simulink model "C_PTES_sim_v2"  (R2025a)
settings: Solver=ode23tb  StartTime=0.0  StopTime=600
PreLoadFcn:
  | Load_Maps
InitFcn:
  | A_init_compressor
StopFcn:
  | % AB_plotHX
  | % AB_plotmap
model workspace (MAT data in the model file):
  Step_time = 1000
  step_time = 200
values from neighbouring files (symbols this model uses):
  DeltaW = 0    [A_init_compressor.m]    (also in B_init_compressor.m = input('Power change: '))
  Ki_tau = 23.1297    [A_init_compressor.m]    (also in B_init_compressor.m = 0.1)
  Kp_tau = 289.6844    [A_init_compressor.m]    (also in B_init_compressor.m = 1)
  omega_step = 376    [A_init_compressor.m]
  stepping_time = 100000    [A_init_compressor.m]    (also in B_init_compressor.m = input('Step time:'))
  tchange = 100000    [A_init_compressor.m]
undefined symbols (not defined in the file or in its folder): z_Qlty_CO2
libraries: simulink_extras x17, slpidlib x9
(part 2 of 3)

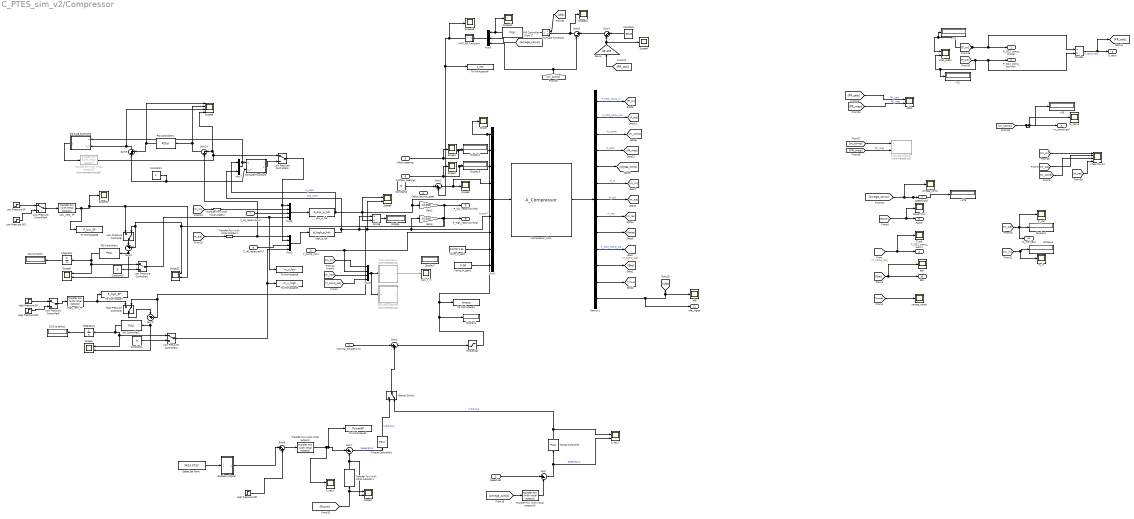
== system C_PTES_sim_v2/Compressor ==
  nominal_torque(N.m) : Inport
  Speed Set : Inport  Port=2
  T_comp_in(K) : Inport  Port=3
  Delta_recycle_open : Inport  Port=4
  Inflow_opening : Inport  Port=5
  Outflow_opening : Inport  Port=6
  T_LP_reservior(K) : Inport  Port=7
  T_HP_reservior(K) : Inport  Port=8
  CO2 to tanks : Display
  CO2 to tanks1 : Display
  Calc Inlet Temp : MATLAB Function  Commented=on  TreatAsAtomicUnit=on
  Compressor_Func : S-Function  FunctionName=A_Compressor  Parameters=Param  SFunctionDeploymentMode=off  EnableBusSupport=off
  Constant : Constant  Value=-89.45
  Constant1 : Constant
  Constant2 : Constant  Value=0
  Constant3 : Constant  Value=0
  Constant4 : Constant  Value=0
  Cool Recycle/Inlet : MATLAB Function  Commented=on  TreatAsAtomicUnit=on
  Demux1 : Demux  Outputs=13
  Display{,2..7} (7 alike) : Display
  Divide : Product  Inputs=*/
  Divide1 : Product  Inputs=/*
  Gain2 : Gain  Gain=1/1000
  Gain3 : Gain  Gain=1/1000
  Gain4 : Gain  Gain=45.455
  High Pressure Controller : ManualSwitch  CurrentSetting=0
  High Pressure SP : Step  Time=tchange  Before=7404*2.502  After=2300*2.34  SampleTime=0
  High Pressure SP1 : Step  Time=5000000  After=DeltaW  SampleTime=0
  High Pressure SP2 : Step  Time=tchange  Before=1100*2.3  After=1100*2.3  SampleTime=0
  High_vent_TF : simulink_extras/Additional Linear/Transfer Fcn (with initial outputs)  N=[1]  D=[10 1]  Y0=7404*2.502  U0=7404*2.502
  Inlet_press : Scope  NumInputPorts=2
      settings: ActiveDisplayYMinimum=-1201.3430582263272  ActiveDisplayYMaximum=21212.950352909458  DataLoggingVariableName=ScopeData18
  Integrator : Integrator
  Integrator1 : Integrator
  Low Pressure Controller : ManualSwitch  CurrentSetting=0
  Low Pressure Controller{1..5} (5 alike) : ManualSwitch
  Low Pressure SP : Step  Time=tchange  Before=7404  After=2300  SampleTime=0
  Low Pressure SP1 : Step  Time=tchange  Before=1100  After=1100  SampleTime=0
  Low_vent_TF : simulink_extras/Additional Linear/Transfer Fcn (with initial outputs)  N=[1]  D=[10 1]  Y0=7404  U0=7404
  MATLAB Function : MATLAB Function  Commented=on  TreatAsAtomicUnit=on
  MATLAB Function1 : MATLAB Function  TreatAsAtomicUnit=on
  MATLAB Function2 : MATLAB Function  TreatAsAtomicUnit=on
  MATLAB Function3 : MATLAB Function  TreatAsAtomicUnit=on
  MATLAB Function4 : MATLAB Function  TreatAsAtomicUnit=on
  Manual Switch : ManualSwitch  CurrentSetting=0
  Mux1 : Mux  Inputs=9
  Mux2 : Mux
  Mux3 : Mux
  Mux5 : Mux  Inputs=3
  Mux6 : Mux
  Mux7 : Mux  Inputs=2
  PID Controller : slpidlib/PID Controller  Controller=PI  Form=Parallel  TimeDomain=Continuous-time  UseExternalTs=off  SampleTime=-1  IntegratorMethod=Forward Euler  FilterMethod=Forward Euler  ControllerParametersSource=internal  P=0.005  I=0.0002  UseKiTs=off  D=0  UseExternalDerivativeSource=off  N=100  UseFilter=on  TunerSelectOption=Transfer Function Based (PID Tuner App)  InitialConditionSource=internal  InitialConditionForIntegrator=0  InitialConditionForFilter=0  DifferentiatorICPrevScaledInput=0  ExternalReset=none  TrackingMode=off  Kt=1  LimitOutput=on  SatLimitsSource=internal  UpperSaturationLimit=1  LowerSaturationLimit=0  LinearizeAsGain=on  AntiWindupMode=back-calculation  Kb=10  LimitIntegrator=on  UpperIntegratorSaturationLimit=inf  LowerIntegratorSaturationLimit=-inf  POutMin=[]  POutMax=[]  IOutMin=[]  IOutMax=[]  DOutMin=[]  DOutMax=[]  NOutMin=[]  NOutMax=[]  SumOutMin=[]  SumOutMax=[]  SaturationOutMin=[]  SaturationOutMax=[]  PParamMin=[]  PParamMax=[]  IParamMin=[]  IParamMax=[]  DParamMin=[]  DParamMax=[]  NParamMin=[]  NParamMax=[]  KbParamMin=[]  KbParamMax=[]  KtParamMin=[]  KtParamMax=[]  KbOutMin=[]  KbOutMax=[]  KtOutMin=[]  KtOutMax=[]  IntegratorOutMin=[]  IntegratorOutMax=[]  FilterOutMin=[]  FilterOutMax=[]  SumI1OutMin=[]  SumI1OutMax=[]  SumI2OutMin=[]  SumI2OutMax=[]  SumI3OutMin=[]  SumI3OutMax=[]  SumI4OutMin=[]  SumI4OutMax=[]  SumDOutMin=[]  SumDOutMax=[]  DifferentiatorOutMin=[]  DifferentiatorOutMax=[]  FilterDiffOutCoefMin=[]  FilterDiffOutCoefMax=[]  ReciprocalOutMin=[]  ReciprocalOutMax=[]  SumDenOutMin=[]  SumDenOutMax=[]  SumNumOutMin=[]  SumNumOutMax=[]  DivideOutMin=[]  DivideOutMax=[]  UdiffTsProdOutMin=[]  UdiffTsProdOutMax=[]  NTsProdOutMin=[]  NTsProdOutMax=[]  UintegralTsProdOutMin=[]  UintegralTsProdOutMax=[]  UngainTsProdOutMin=[]  UngainTsProdOutMax=[]  ClampingZeroOutDataTypeStr=Inherit: Inherit via back propagation  ClampingZeroOutMin=[]  ClampingZeroOutMax=[]  FilterDenConstantOutDataTypeStr=Inherit: Inherit via back propagation  FilterDenConstantOutMin=[]  FilterDenConstantOutMax=[]  PCopyOutDataTypeStr=Inherit: Inherit via back propagation  PCopyOutMin=[]  PCopyOutMax=[]  NCopyOutDataTypeStr=Inherit: Inherit via back propagation  NCopyOutMin=[]  NCopyOutMax=[]  IntegratorContinuousStateAttributes=''  IntegratorStateMustResolveToSignalObject=off  IntegratorRTWStateStorageClass=Auto  FilterContinuousStateAttributes=''  FilterStateMustResolveToSignalObject=off  FilterRTWStateStorageClass=Auto  ParallelPVariant=InternalParameters  IdealPVariant=Disabled  IVariant=InternalParameters  DVariant=Disabled  IntegratorVariant=Continuous  SatVariant=Enabled  AWVariant=BackCalculation  PCopyVariant=Disabled  TRVariant=Disabled  FdbkBlocksVariant=Forward  IdealPFdbkVariant=Disabled  SatFdbkVariant=Disabled  DerivativeFilterVariant=Disabled  NVariant=Disabled  NCopyVariant=Disabled_SignalSpec  FilterICVariant=Disabled  IntegratorICVariant=InternalICs  ExternalResetVariant=Disabled  TRSumVariant=Passthrough  SumFdbkVariant=Disabled  SumVariant=Sum_PI  TsampFilterVariant=InternalTs  TsampNgainVariant=Passthrough  TsampIntegralVariant=Disabled_SignalSpec  ExternalSaturationOutDataTypeStr=Inherit: Same as second input  DerivativeSourceVariant=Disabled  PreIntVariant=InternalPreInt
  PID Controller1 : slpidlib/PID Controller  Controller=PI  Form=Parallel  TimeDomain=Continuous-time  UseExternalTs=off  SampleTime=-1  IntegratorMethod=Forward Euler  FilterMethod=Forward Euler  ControllerParametersSource=internal  P=0.005  I=0.003  UseKiTs=off  D=0  UseExternalDerivativeSource=off  N=100  UseFilter=on  TunerSelectOption=Transfer Function Based (PID Tuner App)  InitialConditionSource=internal  InitialConditionForIntegrator=0  InitialConditionForFilter=0  DifferentiatorICPrevScaledInput=0  ExternalReset=none  TrackingMode=off  Kt=1  LimitOutput=off  SatLimitsSource=internal  UpperSaturationLimit=50  LowerSaturationLimit=-50  LinearizeAsGain=on  AntiWindupMode=none  Kb=1  LimitIntegrator=off  UpperIntegratorSaturationLimit=inf  LowerIntegratorSaturationLimit=-inf  POutMin=[]  POutMax=[]  IOutMin=[]  IOutMax=[]  DOutMin=[]  DOutMax=[]  NOutMin=[]  NOutMax=[]  SumOutMin=[]  SumOutMax=[]  SaturationOutMin=[]  SaturationOutMax=[]  PParamMin=[]  PParamMax=[]  IParamMin=[]  IParamMax=[]  DParamMin=[]  DParamMax=[]  NParamMin=[]  NParamMax=[]  KbParamMin=[]  KbParamMax=[]  KtParamMin=[]  KtParamMax=[]  KbOutMin=[]  KbOutMax=[]  KtOutMin=[]  KtOutMax=[]  IntegratorOutMin=[]  IntegratorOutMax=[]  FilterOutMin=[]  FilterOutMax=[]  SumI1OutMin=[]  SumI1OutMax=[]  SumI2OutMin=[]  SumI2OutMax=[]  SumI3OutMin=[]  SumI3OutMax=[]  SumI4OutMin=[]  SumI4OutMax=[]  SumDOutMin=[]  SumDOutMax=[]  DifferentiatorOutMin=[]  DifferentiatorOutMax=[]  FilterDiffOutCoefMin=[]  FilterDiffOutCoefMax=[]  ReciprocalOutMin=[]  ReciprocalOutMax=[]  SumDenOutMin=[]  SumDenOutMax=[]  SumNumOutMin=[]  SumNumOutMax=[]  DivideOutMin=[]  DivideOutMax=[]  UdiffTsProdOutMin=[]  UdiffTsProdOutMax=[]  NTsProdOutMin=[]  NTsProdOutMax=[]  UintegralTsProdOutMin=[]  UintegralTsProdOutMax=[]  UngainTsProdOutMin=[]  UngainTsProdOutMax=[]  ClampingZeroOutDataTypeStr=Inherit: Inherit via back propagation  ClampingZeroOutMin=[]  ClampingZeroOutMax=[]  FilterDenConstantOutDataTypeStr=Inherit: Inherit via back propagation  FilterDenConstantOutMin=[]  FilterDenConstantOutMax=[]  PCopyOutDataTypeStr=Inherit: Inherit via back propagation  PCopyOutMin=[]  PCopyOutMax=[]  NCopyOutDataTypeStr=Inherit: Inherit via back propagation  NCopyOutMin=[]  NCopyOutMax=[]  IntegratorContinuousStateAttributes=''  IntegratorStateMustResolveToSignalObject=off  IntegratorRTWStateStorageClass=Auto  FilterContinuousStateAttributes=''  FilterStateMustResolveToSignalObject=off  FilterRTWStateStorageClass=Auto  ParallelPVariant=InternalParameters  IdealPVariant=Disabled  IVariant=InternalParameters  DVariant=Disabled  IntegratorVariant=Continuous  SatVariant=Disabled  AWVariant=Passthrough  PCopyVariant=Disabled  TRVariant=Disabled  FdbkBlocksVariant=Forward  IdealPFdbkVariant=Disabled  SatFdbkVariant=Disabled  DerivativeFilterVariant=Disabled  NVariant=Disabled  NCopyVariant=Disabled_SignalSpec  FilterICVariant=Disabled  IntegratorICVariant=InternalICs  ExternalResetVariant=Disabled  TRSumVariant=Passthrough  SumFdbkVariant=Disabled  SumVariant=Sum_PI  TsampFilterVariant=InternalTs  TsampNgainVariant=Passthrough  TsampIntegralVariant=Disabled_SignalSpec  ExternalSaturationOutDataTypeStr=Inherit: Same as second input  DerivativeSourceVariant=Disabled  PreIntVariant=InternalPreInt
  PID Controller2 : slpidlib/PID Controller  Controller=PI  Form=Parallel  TimeDomain=Continuous-time  UseExternalTs=off  SampleTime=-1  IntegratorMethod=Forward Euler  FilterMethod=Forward Euler  ControllerParametersSource=internal  P=0.005  I=0.003  UseKiTs=off  D=0  UseExternalDerivativeSource=off  N=100  UseFilter=on  TunerSelectOption=Transfer Function Based (PID Tuner App)  InitialConditionSource=internal  InitialConditionForIntegrator=0  InitialConditionForFilter=0  DifferentiatorICPrevScaledInput=0  ExternalReset=none  TrackingMode=off  Kt=1  LimitOutput=off  SatLimitsSource=internal  UpperSaturationLimit=50  LowerSaturationLimit=-50  LinearizeAsGain=on  AntiWindupMode=back-calculation  Kb=1  LimitIntegrator=off  UpperIntegratorSaturationLimit=inf  LowerIntegratorSaturationLimit=-inf  POutMin=[]  POutMax=[]  IOutMin=[]  IOutMax=[]  DOutMin=[]  DOutMax=[]  NOutMin=[]  NOutMax=[]  SumOutMin=[]  SumOutMax=[]  SaturationOutMin=[]  SaturationOutMax=[]  PParamMin=[]  PParamMax=[]  IParamMin=[]  IParamMax=[]  DParamMin=[]  DParamMax=[]  NParamMin=[]  NParamMax=[]  KbParamMin=[]  KbParamMax=[]  KtParamMin=[]  KtParamMax=[]  KbOutMin=[]  KbOutMax=[]  KtOutMin=[]  KtOutMax=[]  IntegratorOutMin=[]  IntegratorOutMax=[]  FilterOutMin=[]  FilterOutMax=[]  SumI1OutMin=[]  SumI1OutMax=[]  SumI2OutMin=[]  SumI2OutMax=[]  SumI3OutMin=[]  SumI3OutMax=[]  SumI4OutMin=[]  SumI4OutMax=[]  SumDOutMin=[]  SumDOutMax=[]  DifferentiatorOutMin=[]  DifferentiatorOutMax=[]  FilterDiffOutCoefMin=[]  FilterDiffOutCoefMax=[]  ReciprocalOutMin=[]  ReciprocalOutMax=[]  SumDenOutMin=[]  SumDenOutMax=[]  SumNumOutMin=[]  SumNumOutMax=[]  DivideOutMin=[]  DivideOutMax=[]  UdiffTsProdOutMin=[]  UdiffTsProdOutMax=[]  NTsProdOutMin=[]  NTsProdOutMax=[]  UintegralTsProdOutMin=[]  UintegralTsProdOutMax=[]  UngainTsProdOutMin=[]  UngainTsProdOutMax=[]  ClampingZeroOutDataTypeStr=Inherit: Inherit via back propagation  ClampingZeroOutMin=[]  ClampingZeroOutMax=[]  FilterDenConstantOutDataTypeStr=Inherit: Inherit via back propagation  FilterDenConstantOutMin=[]  FilterDenConstantOutMax=[]  PCopyOutDataTypeStr=Inherit: Inherit via back propagation  PCopyOutMin=[]  PCopyOutMax=[]  NCopyOutDataTypeStr=Inherit: Inherit via back propagation  NCopyOutMin=[]  NCopyOutMax=[]  IntegratorContinuousStateAttributes=''  IntegratorStateMustResolveToSignalObject=off  IntegratorRTWStateStorageClass=Auto  FilterContinuousStateAttributes=''  FilterStateMustResolveToSignalObject=off  FilterRTWStateStorageClass=Auto  ParallelPVariant=InternalParameters  IdealPVariant=Disabled  IVariant=InternalParameters  DVariant=Disabled  IntegratorVariant=Continuous  SatVariant=Disabled  AWVariant=Passthrough  PCopyVariant=Disabled  TRVariant=Disabled  FdbkBlocksVariant=Forward  IdealPFdbkVariant=Disabled  SatFdbkVariant=Disabled  DerivativeFilterVariant=Disabled  NVariant=Disabled  NCopyVariant=Disabled_SignalSpec  FilterICVariant=Disabled  IntegratorICVariant=InternalICs  ExternalResetVariant=Disabled  TRSumVariant=Passthrough  SumFdbkVariant=Disabled  SumVariant=Sum_PI  TsampFilterVariant=InternalTs  TsampNgainVariant=Passthrough  TsampIntegralVariant=Disabled_SignalSpec  ExternalSaturationOutDataTypeStr=Inherit: Same as second input  DerivativeSourceVariant=Disabled  PreIntVariant=InternalPreInt
  PID Controller3 : slpidlib/PID Controller  Controller=PID  Form=Parallel  TimeDomain=Continuous-time  UseExternalTs=off  SampleTime=-1  IntegratorMethod=Forward Euler  FilterMethod=Forward Euler  ControllerParametersSource=internal  P=2  I=0.5  UseKiTs=off  D=0  UseExternalDerivativeSource=off  N=100  UseFilter=on  TunerSelectOption=Transfer Function Based (PID Tuner App)  InitialConditionSource=internal  InitialConditionForIntegrator=0  InitialConditionForFilter=0  DifferentiatorICPrevScaledInput=0  ExternalReset=none  TrackingMode=off  Kt=1  LimitOutput=on  SatLimitsSource=internal  UpperSaturationLimit=5  LowerSaturationLimit=-1  LinearizeAsGain=on  AntiWindupMode=back-calculation  Kb=1  LimitIntegrator=off  UpperIntegratorSaturationLimit=inf  LowerIntegratorSaturationLimit=-inf  POutMin=[]  POutMax=[]  IOutMin=[]  IOutMax=[]  DOutMin=[]  DOutMax=[]  NOutMin=[]  NOutMax=[]  SumOutMin=[]  SumOutMax=[]  SaturationOutMin=[]  SaturationOutMax=[]  PParamMin=[]  PParamMax=[]  IParamMin=[]  IParamMax=[]  DParamMin=[]  DParamMax=[]  NParamMin=[]  NParamMax=[]  KbParamMin=[]  KbParamMax=[]  KtParamMin=[]  KtParamMax=[]  KbOutMin=[]  KbOutMax=[]  KtOutMin=[]  KtOutMax=[]  IntegratorOutMin=[]  IntegratorOutMax=[]  FilterOutMin=[]  FilterOutMax=[]  SumI1OutMin=[]  SumI1OutMax=[]  SumI2OutMin=[]  SumI2OutMax=[]  SumI3OutMin=[]  SumI3OutMax=[]  SumI4OutMin=[]  SumI4OutMax=[]  SumDOutMin=[]  SumDOutMax=[]  DifferentiatorOutMin=[]  DifferentiatorOutMax=[]  FilterDiffOutCoefMin=[]  FilterDiffOutCoefMax=[]  ReciprocalOutMin=[]  ReciprocalOutMax=[]  SumDenOutMin=[]  SumDenOutMax=[]  SumNumOutMin=[]  SumNumOutMax=[]  DivideOutMin=[]  DivideOutMax=[]  UdiffTsProdOutMin=[]  UdiffTsProdOutMax=[]  NTsProdOutMin=[]  NTsProdOutMax=[]  UintegralTsProdOutMin=[]  UintegralTsProdOutMax=[]  UngainTsProdOutMin=[]  UngainTsProdOutMax=[]  ClampingZeroOutDataTypeStr=Inherit: Inherit via back propagation  ClampingZeroOutMin=[]  ClampingZeroOutMax=[]  FilterDenConstantOutDataTypeStr=Inherit: Inherit via back propagation  FilterDenConstantOutMin=[]  FilterDenConstantOutMax=[]  PCopyOutDataTypeStr=Inherit: Inherit via back propagation  PCopyOutMin=[]  PCopyOutMax=[]  NCopyOutDataTypeStr=Inherit: Inherit via back propagation  NCopyOutMin=[]  NCopyOutMax=[]  IntegratorContinuousStateAttributes=''  IntegratorStateMustResolveToSignalObject=off  IntegratorRTWStateStorageClass=Auto  FilterContinuousStateAttributes=''  FilterStateMustResolveToSignalObject=off  FilterRTWStateStorageClass=Auto  ParallelPVariant=InternalParameters  IdealPVariant=Disabled  IVariant=InternalParameters  DVariant=InternalParameters  IntegratorVariant=Continuous  SatVariant=Enabled  AWVariant=BackCalculation  PCopyVariant=Disabled  TRVariant=Disabled  FdbkBlocksVariant=Forward  IdealPFdbkVariant=Disabled  SatFdbkVariant=Disabled  DerivativeFilterVariant=ContFilter  NVariant=InternalParameters  NCopyVariant=Disabled  FilterICVariant=InternalICsFilter  IntegratorICVariant=InternalICs  ExternalResetVariant=Disabled  TRSumVariant=Passthrough  SumFdbkVariant=Disabled  SumVariant=Sum_PID  TsampFilterVariant=InternalTs  TsampNgainVariant=Passthrough  TsampIntegralVariant=Disabled_SignalSpec  ExternalSaturationOutDataTypeStr=Inherit: Same as second input  DerivativeSourceVariant=ErrorSignal  PreIntVariant=InternalPreInt
  Power(kW) : Scope
      settings: ActiveDisplayYMinimum=9621.7825106762266  ActiveDisplayYMaximum=9623.07314717155  DataLoggingSaveFormat=Array
  Scope{,1..3,9..11,13..14} (9 alike) : Scope
      Scope settings: ActiveDisplayYMinimum=7159.4982132893756  ActiveDisplayYMaximum=32715.546490584897  DataLoggingVariableName=ScopeData2
      Scope1 settings: ActiveDisplayYMinimum=0.66249029672546578  ActiveDisplayYMaximum=1.037501078141615  DataLoggingVariableName=ScopeData3
      Scope10 settings: ActiveDisplayYMinimum=-0.1487440658614268  ActiveDisplayYMaximum=0.0708941770326301  DataLoggingVariableName=ScopeData2
      Scope11 settings: ActiveDisplayYMinimum=-1  ActiveDisplayYMaximum=1  DataLoggingVariableName=ScopeData3
      Scope13 settings: ActiveDisplayYMinimum=7403.9999999999982  ActiveDisplayYMaximum=7404.0000000000036  DataLoggingVariableName=ScopeData63
      Scope14 settings: ActiveDisplayYMinimum=-62.947751511362974  ActiveDisplayYMaximum=-19.709497965627289  DataLoggingVariableName=ScopeData86
      Scope2 settings: ActiveDisplayYMinimum=0.43749999999999889  ActiveDisplayYMaximum=1.0625000000000007  DataLoggingVariableName=ScopeData4
      Scope3 settings: ActiveDisplayYMinimum=-4.9775352924503617E-5  ActiveDisplayYMaximum=2.2984047573706729E-5  DataLoggingVariableName=ScopeData4
      Scope9 settings: ActiveDisplayYMinimum=34.362516239027393  ActiveDisplayYMaximum=130.4282542390518
  Scope{4..7,12} (5 alike) : Scope  NumInputPorts=2
      Scope12 settings: ActiveDisplayYMinimum=5734.2862269607867  ActiveDisplayYMaximum=17518.250083003895  DataLoggingVariableName=ScopeData41
      Scope4 settings: ActiveDisplayYMinimum=-0.00074119709145113429  ActiveDisplayYMaximum=0.0001840673230964241  DataLoggingVariableName=ScopeData20
      Scope5 settings: ActiveDisplayYMinimum=-1  ActiveDisplayYMaximum=1  DataLoggingVariableName=ScopeData43
      Scope6 settings: ActiveDisplayYMinimum=-1.078293953241016E+6  ActiveDisplayYMaximum=2.0704645579169132E+7
      Scope7 settings: ActiveDisplayYMinimum=9621.7825106762266  ActiveDisplayYMaximum=9623.07314717155  DataLoggingVariableName=ScopeData7
  Scope8 : Scope  NumInputPorts=4
      settings: ActiveDisplayYMinimum=-2.4702730991182236  ActiveDisplayYMaximum=3.070460845323943  DataLoggingVariableName=ScopeData88
  Shutdown Signal : Subsystem
  Speed Set Point : Constant  Value=9623.0732
  Sum : Sum  Inputs=|+-
  Sum{1..2,5,8..9} (5 alike) : Sum  Inputs=|++
  Sum10 : Sum  Inputs=|-+
  Sum3 : Sum  Inputs=|-+
  Sum4 : Sum  Inputs=|-+
  Sum6 : Sum  Inputs=|+-
  Sum7 : Sum  Inputs=|+-
  T_out : Scope
      settings: ActiveDisplayYMinimum=840.98204874336943  ActiveDisplayYMaximum=841.08678779671368  DataLoggingVariableName=ScopeData11  DataLoggingSaveFormat=Array
  To Workspace1 : ToWorkspace  VariableName=torque  SampleTime=-1
      settings: Save2DSignal=2-D array (concatenate along first dimension)
  To Workspace2 : ToWorkspace  VariableName=PowerSP  SampleTime=-1
      settings: Save2DSignal=2-D array (concatenate along first dimension)
  To Workspace3 : ToWorkspace  VariableName=m_v_low  SampleTime=-1
      settings: Save2DSignal=2-D array (concatenate along first dimension)
  To Workspace4 : ToWorkspace  VariableName=z_rec  SampleTime=-1
      settings: Save2DSignal=2-D array (concatenate along first dimension)
  To Workspace5 : ToWorkspace  VariableName=m_v_high  SampleTime=-1
      settings: Save2DSignal=2-D array (concatenate along first dimension)
  To Workspace6 : ToWorkspace  VariableName=P_low_SP  SampleTime=-1
      settings: Save2DSignal=2-D array (concatenate along first dimension)
  To Workspace7 : ToWorkspace  VariableName=P_high_SP  SampleTime=-1
      settings: Save2DSignal=2-D array (concatenate along first dimension)
  Torque Controller : slpidlib/PID Controller  Controller=PI  Form=Parallel  TimeDomain=Continuous-time  UseExternalTs=off  SampleTime=-1  IntegratorMethod=Forward Euler  FilterMethod=Forward Euler  ControllerParametersSource=internal  P=Kp_tau  I=Ki_tau  UseKiTs=off  D=0  UseExternalDerivativeSource=off  N=100  UseFilter=on  TunerSelectOption=Transfer Function Based (PID Tuner App)  InitialConditionSource=internal  InitialConditionForIntegrator=0  InitialConditionForFilter=0  DifferentiatorICPrevScaledInput=0  ExternalReset=none  TrackingMode=off  Kt=1  LimitOutput=off  SatLimitsSource=internal  UpperSaturationLimit=inf  LowerSaturationLimit=-inf  LinearizeAsGain=on  AntiWindupMode=none  Kb=1  LimitIntegrator=off  UpperIntegratorSaturationLimit=inf  LowerIntegratorSaturationLimit=-inf  POutMin=[]  POutMax=[]  IOutMin=[]  IOutMax=[]  DOutMin=[]  DOutMax=[]  NOutMin=[]  NOutMax=[]  SumOutMin=[]  SumOutMax=[]  SaturationOutMin=[]  SaturationOutMax=[]  PParamMin=[]  PParamMax=[]  IParamMin=[]  IParamMax=[]  DParamMin=[]  DParamMax=[]  NParamMin=[]  NParamMax=[]  KbParamMin=[]  KbParamMax=[]  KtParamMin=[]  KtParamMax=[]  KbOutMin=[]  KbOutMax=[]  KtOutMin=[]  KtOutMax=[]  IntegratorOutMin=[]  IntegratorOutMax=[]  FilterOutMin=[]  FilterOutMax=[]  SumI1OutMin=[]  SumI1OutMax=[]  SumI2OutMin=[]  SumI2OutMax=[]  SumI3OutMin=[]  SumI3OutMax=[]  SumI4OutMin=[]  SumI4OutMax=[]  SumDOutMin=[]  SumDOutMax=[]  DifferentiatorOutMin=[]  DifferentiatorOutMax=[]  FilterDiffOutCoefMin=[]  FilterDiffOutCoefMax=[]  ReciprocalOutMin=[]  ReciprocalOutMax=[]  SumDenOutMin=[]  SumDenOutMax=[]  SumNumOutMin=[]  SumNumOutMax=[]  DivideOutMin=[]  DivideOutMax=[]  UdiffTsProdOutMin=[]  UdiffTsProdOutMax=[]  NTsProdOutMin=[]  NTsProdOutMax=[]  UintegralTsProdOutMin=[]  UintegralTsProdOutMax=[]  UngainTsProdOutMin=[]  UngainTsProdOutMax=[]  ClampingZeroOutDataTypeStr=Inherit: Inherit via back propagation  ClampingZeroOutMin=[]  ClampingZeroOutMax=[]  FilterDenConstantOutDataTypeStr=Inherit: Inherit via back propagation  FilterDenConstantOutMin=[]  FilterDenConstantOutMax=[]  PCopyOutDataTypeStr=Inherit: Inherit via back propagation  PCopyOutMin=[]  PCopyOutMax=[]  NCopyOutDataTypeStr=Inherit: Inherit via back propagation  NCopyOutMin=[]  NCopyOutMax=[]  IntegratorContinuousStateAttributes=''  IntegratorStateMustResolveToSignalObject=off  IntegratorRTWStateStorageClass=Auto  FilterContinuousStateAttributes=''  FilterStateMustResolveToSignalObject=off  FilterRTWStateStorageClass=Auto  ParallelPVariant=InternalParameters  IdealPVariant=Disabled  IVariant=InternalParameters  DVariant=Disabled  IntegratorVariant=Continuous  SatVariant=Disabled  AWVariant=Passthrough  PCopyVariant=Disabled  TRVariant=Disabled  FdbkBlocksVariant=Forward  IdealPFdbkVariant=Disabled  SatFdbkVariant=Disabled  DerivativeFilterVariant=Disabled  NVariant=Disabled  NCopyVariant=Disabled_SignalSpec  FilterICVariant=Disabled  IntegratorICVariant=InternalICs  ExternalResetVariant=Disabled  TRSumVariant=Passthrough  SumFdbkVariant=Disabled  SumVariant=Sum_PI  TsampFilterVariant=InternalTs  TsampNgainVariant=Passthrough  TsampIntegralVariant=Disabled_SignalSpec  ExternalSaturationOutDataTypeStr=Inherit: Same as second input  DerivativeSourceVariant=Disabled  PreIntVariant=InternalPreInt
  Torque Controller1 : slpidlib/PID Controller  Controller=PI  Form=Parallel  TimeDomain=Continuous-time  UseExternalTs=off  SampleTime=-1  IntegratorMethod=Forward Euler  FilterMethod=Forward Euler  ControllerParametersSource=internal  P=0.16  I=0.09  UseKiTs=off  D=0  UseExternalDerivativeSource=off  N=100  UseFilter=on  TunerSelectOption=Transfer Function Based (PID Tuner App)  InitialConditionSource=internal  InitialConditionForIntegrator=3.258241730106488e+04  InitialConditionForFilter=0  DifferentiatorICPrevScaledInput=0  ExternalReset=none  TrackingMode=off  Kt=1  LimitOutput=off  SatLimitsSource=internal  UpperSaturationLimit=inf  LowerSaturationLimit=-inf  LinearizeAsGain=on  AntiWindupMode=none  Kb=1  LimitIntegrator=off  UpperIntegratorSaturationLimit=inf  LowerIntegratorSaturationLimit=-inf  POutMin=[]  POutMax=[]  IOutMin=[]  IOutMax=[]  DOutMin=[]  DOutMax=[]  NOutMin=[]  NOutMax=[]  SumOutMin=[]  SumOutMax=[]  SaturationOutMin=[]  SaturationOutMax=[]  PParamMin=[]  PParamMax=[]  IParamMin=[]  IParamMax=[]  DParamMin=[]  DParamMax=[]  NParamMin=[]  NParamMax=[]  KbParamMin=[]  KbParamMax=[]  KtParamMin=[]  KtParamMax=[]  KbOutMin=[]  KbOutMax=[]  KtOutMin=[]  KtOutMax=[]  IntegratorOutMin=[]  IntegratorOutMax=[]  FilterOutMin=[]  FilterOutMax=[]  SumI1OutMin=[]  SumI1OutMax=[]  SumI2OutMin=[]  SumI2OutMax=[]  SumI3OutMin=[]  SumI3OutMax=[]  SumI4OutMin=[]  SumI4OutMax=[]  SumDOutMin=[]  SumDOutMax=[]  DifferentiatorOutMin=[]  DifferentiatorOutMax=[]  FilterDiffOutCoefMin=[]  FilterDiffOutCoefMax=[]  ReciprocalOutMin=[]  ReciprocalOutMax=[]  SumDenOutMin=[]  SumDenOutMax=[]  SumNumOutMin=[]  SumNumOutMax=[]  DivideOutMin=[]  DivideOutMax=[]  UdiffTsProdOutMin=[]  UdiffTsProdOutMax=[]  NTsProdOutMin=[]  NTsProdOutMax=[]  UintegralTsProdOutMin=[]  UintegralTsProdOutMax=[]  UngainTsProdOutMin=[]  UngainTsProdOutMax=[]  ClampingZeroOutDataTypeStr=Inherit: Inherit via back propagation  ClampingZeroOutMin=[]  ClampingZeroOutMax=[]  FilterDenConstantOutDataTypeStr=Inherit: Inherit via back propagation  FilterDenConstantOutMin=[]  FilterDenConstantOutMax=[]  PCopyOutDataTypeStr=Inherit: Inherit via back propagation  PCopyOutMin=[]  PCopyOutMax=[]  NCopyOutDataTypeStr=Inherit: Inherit via back propagation  NCopyOutMin=[]  NCopyOutMax=[]  IntegratorContinuousStateAttributes=''  IntegratorStateMustResolveToSignalObject=off  IntegratorRTWStateStorageClass=Auto  FilterContinuousStateAttributes=''  FilterStateMustResolveToSignalObject=off  FilterRTWStateStorageClass=Auto  ParallelPVariant=InternalParameters  IdealPVariant=Disabled  IVariant=InternalParameters  DVariant=Disabled  IntegratorVariant=Continuous  SatVariant=Disabled  AWVariant=Passthrough  PCopyVariant=Disabled  TRVariant=Disabled  FdbkBlocksVariant=Forward  IdealPFdbkVariant=Disabled  SatFdbkVariant=Disabled  DerivativeFilterVariant=Disabled  NVariant=Disabled  NCopyVariant=Disabled_SignalSpec  FilterICVariant=Disabled  IntegratorICVariant=InternalICs  ExternalResetVariant=Disabled  TRSumVariant=Passthrough  SumFdbkVariant=Disabled  SumVariant=Sum_PI  TsampFilterVariant=InternalTs  TsampNgainVariant=Passthrough  TsampIntegralVariant=Disabled_SignalSpec  ExternalSaturationOutDataTypeStr=Inherit: Same as second input  DerivativeSourceVariant=Disabled  PreIntVariant=InternalPreInt
  Torque Sat : Saturate  UpperLimit=4.2570e4  LowerLimit=0
  Transfer Fcn (with initial outputs) : simulink_extras/Additional Linear/Transfer Fcn (with initial outputs)  N=[1]  D="[1  1]"  Y0=9623.0732  U0=0
  Transfer Fcn (with initial outputs)1 : simulink_extras/Additional Linear/Transfer Fcn (with initial outputs)  N=[1]  D="[1  1]"  Y0=9623.0732  U0=0
  Transfer Fcn (with initial outputs)2 : simulink_extras/Additional Linear/Transfer Fcn (with initial outputs)  Commented=through  N=[1]  D="[1  1]"  Y0=53.3769  U0=0
  Transfer Fcn (with initial outputs)3 : simulink_extras/Additional Linear/Transfer Fcn (with initial outputs)  N=[1]  D="[1  1]"  Y0=376  U0=0
  Transfer Fcn (with initial states) : simulink_extras/Additional Linear/Transfer Fcn (with initial states)  N=[1]  D="[1  1]"  X0=53.0908043651412
  Transfer Fcn (with initial states)1 : simulink_extras/Additional Linear/Transfer Fcn (with initial states)  N=[1]  D="[1  1]"  X0=53.0908043651412
  Valve_in_gain : Constant  Value=0.1071*1.34
  Valve_in_gain1 : Constant  Value=0.08
  calc_t_in : Scope
      settings: ActiveDisplayYMinimum=-1  ActiveDisplayYMaximum=1  DataLoggingVariableName=ScopeData22  DataLoggingSaveFormat=Array
  eta : Scope
      settings: ActiveDisplayYMinimum=0.058346045029937676  ActiveDisplayYMaximum=0.974885594730561  DataLoggingVariableName=ScopeData12  DataLoggingSaveFormat=Array
  high_p_hdr : S-Function  FunctionName=A_high_p_hdr  Parameters=Param  SFunctionDeploymentMode=off  EnableBusSupport=off
  idle : Scope
      settings: ActiveDisplayYMinimum=-0.12499999999999997  ActiveDisplayYMaximum=1.125  DataLoggingVariableName=ScopeData21  DataLoggingSaveFormat=Array
  idle1 : Scope  NumInputPorts=2
      settings: ActiveDisplayYMinimum=0.94027654878005018  ActiveDisplayYMaximum=1.1257908746996972  DataLoggingVariableName=ScopeData40
  low_p_hdr : S-Function  FunctionName=A_low_p_hdr  Parameters=Param  SFunctionDeploymentMode=off  EnableBusSupport=off
  m_comp : Scope
      settings: ActiveDisplayYMinimum=-6.4294152227829491  ActiveDisplayYMaximum=57.864737008156951  DataLoggingVariableName=ScopeData13  DataLoggingSaveFormat=Array
  m_in : Scope
      settings: ActiveDisplayYMinimum=-5.7642251489523835  ActiveDisplayYMaximum=51.878026340571459  DataLoggingVariableName=ScopeData14
  m_out : Scope
      settings: ActiveDisplayYMinimum=-1.9413639664669944  ActiveDisplayYMaximum=2.9528309069791945  DataLoggingVariableName=ScopeData2
  mass flows1 : Scope  NumInputPorts=4
      settings: ActiveDisplayYMinimum=-6.6752308438687669  ActiveDisplayYMaximum=60.077077594818917  DataLoggingVariableName=ScopeData16  DataLoggingSaveFormat=Array
  omega_comp : Scope
      settings: ActiveDisplayYMinimum=8.3712039774254627  ActiveDisplayYMaximum=10.897406611126089  DataLoggingVariableName=ScopeData17
  t_rec1 : Scope  NumInputPorts=2
      settings: ActiveDisplayYMinimum=-0.00059724971531247353  ActiveDisplayYMaximum=0.00016704312745400825  DataLoggingVariableName=ScopeData87  DataLoggingSaveFormat=Array
  t_rec2 : Scope  NumInputPorts=2
      settings: ActiveDisplayYMinimum=-1202.88415  ActiveDisplayYMaximum=10825.957350000002  DataLoggingVariableName=ScopeData24  DataLoggingSaveFormat=Array
  torque_comp : Scope
      settings: ActiveDisplayYMinimum=-3437.51384  ActiveDisplayYMaximum=30937.62455  DataLoggingSaveFormat=Array
  ~22 : Display
  ~379 : Display
  ~55 : Display
  ~7.4 : Display
  P_CO2_comp_in(kPa) : Outport
  P_CO2_comp_out(kPa) : Outport  Port=2
  m_comp(kg/s) : Outport  Port=3
  T_CO2_comp_out(K) : Outport  Port=4
  P_low_reservior(kPa) : Outport  Port=5
  P_high_reservior(kPa) : Outport  Port=6
  Speed(rpm) : Outport  Port=7
  P_ratio : Outport  Port=8
  Power : Outport  Port=9
  Eta : Outport  Port=10
  idle_signal : Outport  Port=11
  m_out(kg/s) : Outport  Port=12
  wires:
  Demux1/10 -> [T_comp_out]  "T_CO2_comp_out"
  Demux1/12 -> [Torque]
  Demux1/6 -> [m_in]  "M_in"
  Demux1/3 -> [m_comp]  "M_comp"
  Demux1/2 -> [P_out]  "P_CO2_comp_out"
  Compressor_Func/1 -> Demux1/1
  Demux1/8 -> [m_rec]  "m_rec"
  Demux1/1 -> [P_in]  "P_CO2_comp_in"
  Demux1/11 -> [Eta]
  Demux1/9 -> [Power]
  Sum/1 -> t_rec1/2, Torque Controller/1  "Speed Error"
  Mux1/1 -> Compressor_Func/1
  Divide/1 -> Display/1
  Mux3/1 -> low_p_hdr/1
  Mux2/1 -> high_p_hdr/1
  Demux1/5 -> [omega_comp]
  Transfer Fcn (with initial states)/1 -> Mux3/2
  Transfer Fcn (with initial states)1/1 -> Sum10/2, Mux2/1
  Gain2/1 -> Low Pressure Controller/2, Sum4/2, Scope12/1, P_low_reservior(kPa)/1
  Demux1/4 -> [PR_map]  "P_ratio"
  Sum2/1 -> Scope3/1, Mux1/4
  Inflow_opening/1 -> Scope1/1, Display2/1, Mux1/2
  Outflow_opening/1 -> Scope2/1, Display3/1, Mux1/3
  T_HP_reservior(K)/1 -> Mux2/3
  T_LP_reservior(K)/1 -> Mux3/3
  Constant/1 -> Sum5/1
  Sum5/1 -> Sum6/1
  Sum6/1 -> MATLAB Function2/2(x), Scope14/1
  Demux1/7 -> [m_out]  "M_out"
  Constant2/1 -> Sum2/1
  Gain4/1 -> Sum5/2, Scope9/1
  PID Controller/1 -> Scope11/1, Mux5/1
  Mux5/1 -> MATLAB Function4/1(u)
  Torque Controller/1 -> Manual Switch/2, t_rec1/1  "T-PID Out"
  Torque Sat/1 -> To Workspace1/1, Scope/1, Mux1/1, Display4/1  "Actual T"
  Demux1/13 -> [idle], idle/1, idle_signal/1
  nominal_torque(N.m)/1 -> Sum1/1
  Speed Set/1 -> Sum/1
  Sum1/1 -> Torque Sat/1
  Divide1/1 -> [PR_calc], P_ratio/1  "P_ratio_calc"
  Mux6/1 -> Cool Recycle/Inlet/1(u), Calc Inlet Temp/1(u)
  Calc Inlet Temp/1(y) -> calc_t_in/1
  MATLAB Function4/1(y) -> To Workspace4/1, Sum2/2, Scope10/1
  PID Controller1/1 -> Scope5/1, Low Pressure Controller1/1, Integrator/1
  Sum4/1 -> Scope5/2, PID Controller1/1
  Integrator/1 -> CO2 to tanks/1
  Low Pressure Controller/1 -> Sum4/1
  [T_comp_out] -> T_out/1, T_CO2_comp_out(K)/1
  [T_comp_out] -> Mux6/4
  [Eta] -> Eta/1, eta/1
  [Torque] -> torque_comp/1
  [Power] -> Power(kW)/1, Power/1
  [m_rec] -> Mux6/3
  [m_comp] -> mass flows1/3
  [m_out] -> mass flows1/2
  [m_out] -> m_out/1, Display6/1, m_out(kg/s)/1
  [m_in] -> m_in/1, Display5/1
  [m_in] -> Mux6/1
  [m_in] -> mass flows1/1
  [m_in] -> Transfer Fcn (with initial states)/1
  [m_out] -> Transfer Fcn (with initial states)1/1
  [omega_comp] -> Transfer Fcn (with initial outputs)3/1
  [omega_comp] -> Mux5/2
  [omega_comp] -> Speed(rpm)/1, ~379/1, omega_comp/1
  [P_in] -> Divide1/1, P_CO2_comp_in(kPa)/1, ~7.4/1, Inlet_press/1
  [P_out] -> ~22/1, Inlet_press/2, Divide1/2, P_CO2_comp_out(kPa)/1
  [PR_calc] -> Gain4/1
  [m_comp] -> Mux5/3, Sum6/2
  [m_comp] -> m_comp/1, m_comp(kg/s)/1, ~55/1
  [PR_map] -> idle1/2  "PR_map"
  [PR_calc] -> idle1/1  "PR_calc"
  [PR_map] -> MATLAB Function/2(y)  "PR_map"
  [m_comp] -> MATLAB Function/1(x)
  Valve_in_gain/1 -> Mux1/8
  Valve_in_gain1/1 -> Mux1/9
  High Pressure Controller/1 -> Sum3/1
  Integrator1/1 -> CO2 to tanks1/1
  Sum3/1 -> PID Controller2/1, Scope4/2
  PID Controller2/1 -> Integrator1/1, Scope4/1, Low Pressure Controller2/1
  Gain3/1 -> Sum3/2, High Pressure Controller/2, P_high_reservior(kPa)/1
  Low Pressure SP/1 -> Low Pressure Controller4/1
  High Pressure SP/1 -> Low Pressure Controller5/1
  Low_vent_TF/1 -> To Workspace6/1, Low Pressure Controller/1, Scope12/2, Scope13/1
  High_vent_TF/1 -> To Workspace7/1, High Pressure Controller/1
  T_comp_in(K)/1 -> Mux6/2, Mux1/7
  [idle] -> MATLAB Function2/1(u)
  MATLAB Function2/1(y) -> PID Controller/1
  Low Pressure Controller1/1 -> To Workspace3/1, Mux3/4
  Constant3/1 -> Low Pressure Controller1/2
  Constant4/1 -> Low Pressure Controller2/2
  Low Pressure Controller2/1 -> Mux2/4, To Workspace5/1
  Mux7/1 -> MATLAB Function3/1(u), MATLAB Function1/1(u)
  high_p_hdr/1 -> Mux7/2, Divide/1, Scope6/2, Gain3/1, Mux1/6  "Out_pres"
  low_p_hdr/1 -> Mux7/1, Divide/2, Scope6/1, Gain2/1, Mux1/5  "In_pres"
  Low Pressure Controller3/1 -> Mux2/2, Mux3/1
  [m_rec] -> mass flows1/4
  [Power] -> Scope7/1, Transfer Fcn (with initial outputs)1/1
  Sum7/1 -> Torque Controller1/1  "Speed Error"
  Torque Controller1/1 -> Manual Switch/1  "T-PID Out"
  Manual Switch/1 -> Sum1/2
  Speed Set Point/1 -> Shutdown Signal/1(In1)
  Shutdown Signal/1(Out1) -> Sum8/1
  Sum8/1 -> Transfer Fcn (with initial outputs)/1
  Transfer Fcn (with initial outputs)1/1 -> Sum7/2, Scope7/2
  High Pressure SP1/1 -> Sum8/2
  Transfer Fcn (with initial outputs)/1 -> t_rec2/1, To Workspace2/1, Sum7/1
  MATLAB Function1/1(y) -> Low Pressure Controller3/2
  Constant1/1 -> Sum9/1, MATLAB Function1/2(z_v)
  MATLAB Function3/1(y) -> Transfer Fcn (with initial outputs)2/1
  Sum10/1 -> Scope8/2, PID Controller3/1
  Sum9/1 -> Scope8/3, MATLAB Function3/2(z_v)
  Transfer Fcn (with initial outputs)2/1 -> Low Pressure Controller3/1, Scope8/4, Sum10/1
  PID Controller3/1 -> Scope8/1, Sum9/2
  Low Pressure SP1/1 -> Low Pressure Controller4/2
  Low Pressure Controller4/1 -> Low_vent_TF/1
  Low Pressure Controller5/1 -> High_vent_TF/1
  High Pressure SP2/1 -> Low Pressure Controller5/2
  Transfer Fcn (with initial outputs)3/1 -> Sum/2

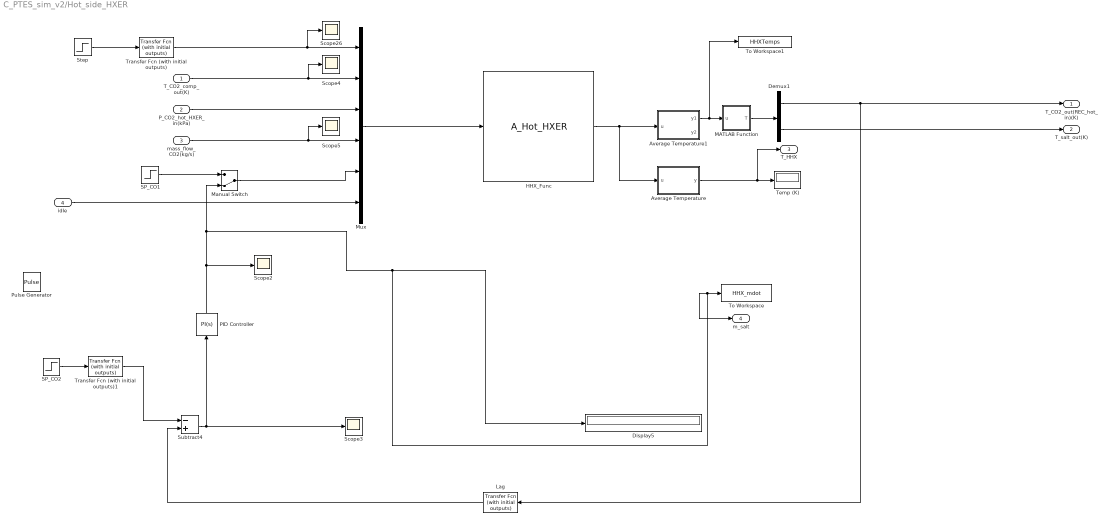
== system C_PTES_sim_v2/Hot_side_HXER ==
  T_CO2_comp_out(K) : Inport
  P_CO2_hot_HXER_in(kPa) : Inport  Port=2
  mass_flow_CO2(kg/s) : Inport  Port=3
  idle : Inport  Port=4
  Average Temperature : MATLAB Function  TreatAsAtomicUnit=on
  Average Temperature1 : MATLAB Function  TreatAsAtomicUnit=on
  Demux1 : Demux  Outputs=2
  Display5 : Display
      settings: Format=long_e
  HHX_Func : S-Function  FunctionName=A_Hot_HXER  Parameters=Param  SFunctionDeploymentMode=off  EnableBusSupport=off
  Lag : simulink_extras/Additional Linear/Transfer Fcn (with initial outputs)  N=[1]  D="[.1  1]"  Y0=425+273.15  U0=0
  MATLAB Function : MATLAB Function  TreatAsAtomicUnit=on
  Manual Switch : ManualSwitch  CurrentSetting=0
  Mux : Mux  Inputs=6
  PID Controller : slpidlib/PID Controller  Controller=PI  Form=Parallel  TimeDomain=Continuous-time  UseExternalTs=off  SampleTime=-1  IntegratorMethod=Forward Euler  FilterMethod=Forward Euler  ControllerParametersSource=internal  P=1  I=0.5  UseKiTs=off  D=0  UseExternalDerivativeSource=off  N=1  UseFilter=on  TunerSelectOption=Transfer Function Based (PID Tuner App)  InitialConditionSource=internal  InitialConditionForIntegrator=0  InitialConditionForFilter=0  DifferentiatorICPrevScaledInput=0  ExternalReset=none  TrackingMode=off  Kt=1  LimitOutput=on  SatLimitsSource=internal  UpperSaturationLimit=1000  LowerSaturationLimit=0  LinearizeAsGain=off  AntiWindupMode=back-calculation  Kb=10  LimitIntegrator=off  UpperIntegratorSaturationLimit=inf  LowerIntegratorSaturationLimit=-inf  POutMin=[]  POutMax=[]  IOutMin=[]  IOutMax=[]  DOutMin=[]  DOutMax=[]  NOutMin=[]  NOutMax=[]  SumOutMin=[]  SumOutMax=[]  SaturationOutMin=[]  SaturationOutMax=[]  PParamMin=[]  PParamMax=[]  IParamMin=[]  IParamMax=[]  DParamMin=[]  DParamMax=[]  NParamMin=[]  NParamMax=[]  KbParamMin=[]  KbParamMax=[]  KtParamMin=[]  KtParamMax=[]  KbOutMin=[]  KbOutMax=[]  KtOutMin=[]  KtOutMax=[]  IntegratorOutMin=[]  IntegratorOutMax=[]  FilterOutMin=[]  FilterOutMax=[]  SumI1OutMin=[]  SumI1OutMax=[]  SumI2OutMin=[]  SumI2OutMax=[]  SumI3OutMin=[]  SumI3OutMax=[]  SumI4OutMin=[]  SumI4OutMax=[]  SumDOutMin=[]  SumDOutMax=[]  DifferentiatorOutMin=[]  DifferentiatorOutMax=[]  FilterDiffOutCoefMin=[]  FilterDiffOutCoefMax=[]  ReciprocalOutMin=[]  ReciprocalOutMax=[]  SumDenOutMin=[]  SumDenOutMax=[]  SumNumOutMin=[]  SumNumOutMax=[]  DivideOutMin=[]  DivideOutMax=[]  UdiffTsProdOutMin=[]  UdiffTsProdOutMax=[]  NTsProdOutMin=[]  NTsProdOutMax=[]  UintegralTsProdOutMin=[]  UintegralTsProdOutMax=[]  UngainTsProdOutMin=[]  UngainTsProdOutMax=[]  ClampingZeroOutDataTypeStr=Inherit: Inherit via back propagation  ClampingZeroOutMin=[]  ClampingZeroOutMax=[]  FilterDenConstantOutDataTypeStr=Inherit: Inherit via back propagation  FilterDenConstantOutMin=[]  FilterDenConstantOutMax=[]  PCopyOutDataTypeStr=Inherit: Inherit via back propagation  PCopyOutMin=[]  PCopyOutMax=[]  NCopyOutDataTypeStr=Inherit: Inherit via back propagation  NCopyOutMin=[]  NCopyOutMax=[]  IntegratorContinuousStateAttributes=''  IntegratorStateMustResolveToSignalObject=off  IntegratorRTWStateStorageClass=Auto  FilterContinuousStateAttributes=''  FilterStateMustResolveToSignalObject=off  FilterRTWStateStorageClass=Auto  ParallelPVariant=InternalParameters  IdealPVariant=Disabled  IVariant=InternalParameters  DVariant=Disabled  IntegratorVariant=Continuous  SatVariant=Enabled  AWVariant=BackCalculation  PCopyVariant=Disabled  TRVariant=Disabled  FdbkBlocksVariant=Forward  IdealPFdbkVariant=Disabled  SatFdbkVariant=Disabled  DerivativeFilterVariant=Disabled  NVariant=Disabled  NCopyVariant=Disabled_SignalSpec  FilterICVariant=Disabled  IntegratorICVariant=InternalICs  ExternalResetVariant=Disabled  TRSumVariant=Passthrough  SumFdbkVariant=Disabled  SumVariant=Sum_PI  TsampFilterVariant=InternalTs  TsampNgainVariant=Passthrough  TsampIntegralVariant=Disabled_SignalSpec  ExternalSaturationOutDataTypeStr=Inherit: Same as second input  DerivativeSourceVariant=Disabled  PreIntVariant=InternalPreInt
  Pulse Generator : DiscretePulseGenerator  PulseType=Time based  Period=6000  PulseWidth=50  PhaseDelay=100
  SP_CO1 : Step  Time=5000  After=0  SampleTime=0
  SP_CO2 : Step  Time=tchange  Before=425+273.15  After=300+273.15  SampleTime=0
  Scope{2..5,26} (5 alike) : Scope
      Scope2 settings: ActiveDisplayYMinimum=42.789048961394684  ActiveDisplayYMaximum=42.792395745185487
      Scope26 settings: ActiveDisplayYMinimum=-1  ActiveDisplayYMaximum=1  DataLoggingVariableName=ScopeData4
      Scope3 settings: ActiveDisplayYMinimum=-371.71225223306891  ActiveDisplayYMaximum=41.918565740840968  DataLoggingVariableName=ScopeData2
      Scope4 settings: ActiveDisplayYMinimum=305.62905977062007  ActiveDisplayYMaximum=906.319539816441  DataLoggingVariableName=ScopeData3
      Scope5 settings: ActiveDisplayYMinimum=-6.67367893688812  ActiveDisplayYMaximum=60.063110431993096  DataLoggingVariableName=ScopeData2
  Step : Step  Time=tchange  Before=420+273.15  After=295+273.15  SampleTime=0
  Subtract4 : Sum  Inputs=-+
  Temp (K) : Display
  To Workspace : ToWorkspace  VariableName=HHX_mdot  SampleTime=-1
  To Workspace1 : ToWorkspace  VariableName=HHXTemps  SampleTime=-1
      settings: Save2DSignal=2-D array (concatenate along first dimension)
  Transfer Fcn (with initial outputs) : simulink_extras/Additional Linear/Transfer Fcn (with initial outputs)  N=[1]  D="[5  1]"  Y0=420+273.15  U0=0
  Transfer Fcn (with initial outputs)1 : simulink_extras/Additional Linear/Transfer Fcn (with initial outputs)  N=[1]  D="[5  1]"  Y0=425+273.15  U0=0
  T_CO2_out(REC_hot_in)(K) : Outport
  T_salt_out(K) : Outport  Port=2
  T_HHX : Outport  Port=3
  m_salt : Outport  Port=4
  wires:
  P_CO2_hot_HXER_in(kPa)/1 -> Mux/3
  T_CO2_comp_out(K)/1 -> Scope4/1, Mux/2
  mass_flow_CO2(kg/s)/1 -> Scope5/1, Mux/4
  Step/1 -> Transfer Fcn (with initial outputs)/1
  Subtract4/1 -> PID Controller/1, Scope3/1
  Demux1/1 -> Lag/1, T_CO2_out(REC_hot_in)(K)/1
  Demux1/2 -> T_salt_out(K)/1
  MATLAB Function/1(T) -> Demux1/1
  Mux/1 -> HHX_Func/1
  HHX_Func/1 -> Average Temperature/1(u), Average Temperature1/1(u)
  Average Temperature/1(y) -> T_HHX/1, Temp (K)/1
  idle/1 -> Mux/6
  Average Temperature1/1(y1) -> To Workspace1/1, MATLAB Function/1(u)
  PID Controller/1 -> m_salt/1, To Workspace/1, Display5/1, Manual Switch/2, Scope2/1
  SP_CO2/1 -> Transfer Fcn (with initial outputs)1/1
  SP_CO1/1 -> Manual Switch/1
  Manual Switch/1 -> Mux/5
  Lag/1 -> Subtract4/2
  Transfer Fcn (with initial outputs)/1 -> Scope26/1, Mux/1
  Transfer Fcn (with initial outputs)1/1 -> Subtract4/1

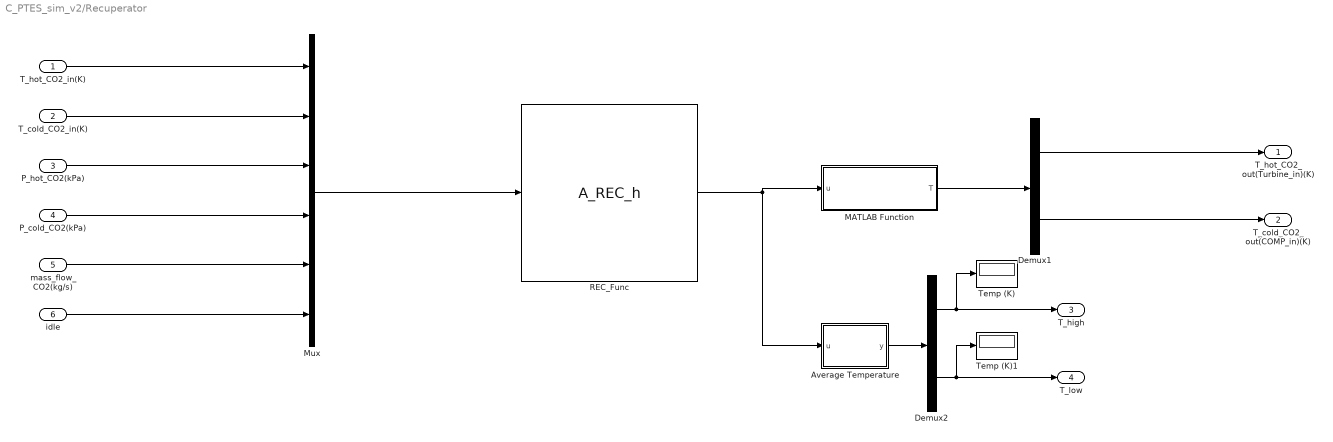
== system C_PTES_sim_v2/Recuperator ==
  T_hot_CO2_in(K) : Inport
  T_cold_CO2_in(K) : Inport  Port=2
  P_hot_CO2(kPa) : Inport  Port=3
  P_cold_CO2(kPa) : Inport  Port=4
  mass_flow_CO2(kg/s) : Inport  Port=5
  idle : Inport  Port=6
  Average Temperature : MATLAB Function  TreatAsAtomicUnit=on
  Demux1 : Demux  Outputs=2
  Demux2 : Demux  Outputs=2
  MATLAB Function : MATLAB Function  TreatAsAtomicUnit=on
  Mux : Mux  Inputs=6
  REC_Func : S-Function  InitFcn=A_init_compressor  FunctionName=A_REC_h  Parameters=Param  SFunctionDeploymentMode=off  EnableBusSupport=off
  Temp (K) : Display
  Temp (K)1 : Display
  T_hot_CO2_out(Turbine_in)(K) : Outport
  T_cold_CO2_out(COMP_in)(K) : Outport  Port=2
  T_high : Outport  Port=3
  T_low : Outport  Port=4
  wires:
  T_cold_CO2_in(K)/1 -> Mux/2
  P_cold_CO2(kPa)/1 -> Mux/4
  P_hot_CO2(kPa)/1 -> Mux/3
  mass_flow_CO2(kg/s)/1 -> Mux/5
  T_hot_CO2_in(K)/1 -> Mux/1
  Mux/1 -> REC_Func/1
  MATLAB Function/1(T) -> Demux1/1
  Demux1/1 -> T_hot_CO2_out(Turbine_in)(K)/1
  Demux1/2 -> T_cold_CO2_out(COMP_in)(K)/1
  REC_Func/1 -> MATLAB Function/1(u), Average Temperature/1(u)
  Average Temperature/1(y) -> Demux2/1
  Demux2/1 -> Temp (K)/1, T_high/1
  Demux2/2 -> T_low/1, Temp (K)1/1
  idle/1 -> Mux/6

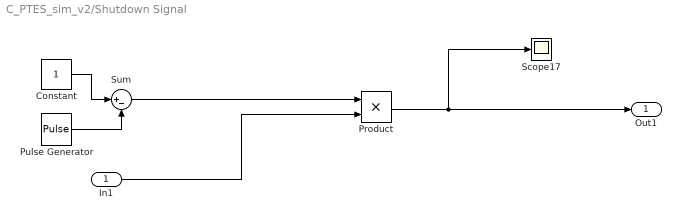
== system C_PTES_sim_v2/Shutdown Signal ==
  In1 : Inport
  Constant : Constant
  Product : Product
  Pulse Generator : DiscretePulseGenerator  PulseType=Time based  Period=4000  PulseWidth=27.5  PhaseDelay=100
  Scope17 : Scope
      settings: ActiveDisplayYMinimum=346.2691444179722  ActiveDisplayYMaximum=643.57770023825037  DataLoggingVariableName=ScopeData23
  Sum : Sum  Inputs=|+-
  Out1 : Outport
  wires:
  Product/1 -> Scope17/1, Out1/1
  In1/1 -> Product/2
  Sum/1 -> Product/1
  Pulse Generator/1 -> Sum/2
  Constant/1 -> Sum/1

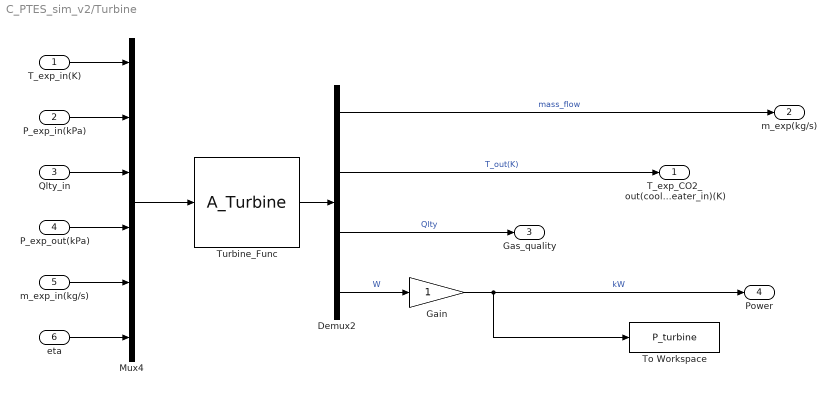
== system C_PTES_sim_v2/Turbine ==
  T_exp_in(K) : Inport
  P_exp_in(kPa) : Inport  Port=2
  Qlty_in : Inport  Port=3
  P_exp_out(kPa) : Inport  Port=4
  m_exp_in(kg/s) : Inport  Port=5
  eta : Inport  Port=6
  Demux2 : Demux
  Gain : Gain
  Mux4 : Mux  Inputs=6
  To Workspace : ToWorkspace  VariableName=P_turbine  SampleTime=-1
      settings: Save2DSignal=2-D array (concatenate along first dimension)
  "Turbine_Func " : S-Function  FunctionName=A_Turbine  Parameters=Param  SFunctionDeploymentMode=off  EnableBusSupport=off
  T_exp_CO2_out(cooler&heater_in)(K) : Outport
  m_exp(kg/s) : Outport  Port=2
  Gas_quality : Outport  Port=3
  Power : Outport  Port=4
  wires:
  Demux2/3 -> Gas_quality/1  "Qlty"
  Demux2/2 -> T_exp_CO2_out(cooler&heater_in)(K)/1  "T_out(K)"
  T_exp_in(K)/1 -> Mux4/1
  Qlty_in/1 -> Mux4/3
  P_exp_in(kPa)/1 -> Mux4/2
  "Turbine_Func "/1 -> Demux2/1
  Demux2/4 -> Gain/1  "W"
  Gain/1 -> Power/1, To Workspace/1  "kW"
  Demux2/1 -> m_exp(kg/s)/1  "mass_flow"
  P_exp_out(kPa)/1 -> Mux4/4
  Mux4/1 -> "Turbine_Func "/1
  m_exp_in(kg/s)/1 -> Mux4/5
  eta/1 -> Mux4/6

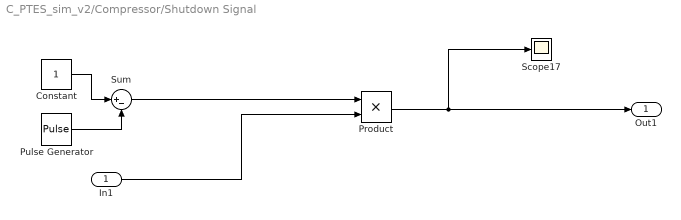
== system C_PTES_sim_v2/Compressor/Shutdown Signal ==
  In1 : Inport
  Constant : Constant
  Product : Product
  Pulse Generator : DiscretePulseGenerator  PulseType=Time based  Amplitude=0  Period=4000  PulseWidth=27.5  PhaseDelay=100
  Scope17 : Scope
      settings: ActiveDisplayYMinimum=346.2691444179722  ActiveDisplayYMaximum=643.57770023825037  DataLoggingVariableName=ScopeData23
  Sum : Sum  Inputs=|+-
  Out1 : Outport
  wires:
  Product/1 -> Scope17/1, Out1/1
  In1/1 -> Product/2
  Sum/1 -> Product/1
  Pulse Generator/1 -> Sum/2
  Constant/1 -> Sum/1

== matlab function C_PTES_sim_v2/Cold_side_HXER/MATLAB Function ==
  data: u input; T output
function T = extract_outlet_temps(u)

n=length(u)/2;

u1=u(1:n);
u2=u(n+1:2*n);

T1=u1(end);
T2=u2(end);
T=[T1,T2];
end

== matlab function C_PTES_sim_v2/Compressor/MATLAB Function2 ==
  data: u input; y output; x input
function y = fcn(u, x)

if u
    y=0;
else
    y=x;
end

== matlab function C_PTES_sim_v2/Compressor/MATLAB Function3 ==
  data: u input; y output; z_v input
function y = fcn(u,z_v)

% Valve_in_gain=0.016009671392157882;
Valve_in_gain=0.0160055850737664*(1+-7.285480376175610e-05);
In_pres=u(1);
Out_pres=u(2);
m_in     = Valve_in_gain*z_v* sqrt(abs(Out_pres - In_pres)) * (Out_pres - In_pres)/abs(Out_pres - In_pres);
y = m_in;

== matlab function C_PTES_sim_v2/Recuperator/MATLAB Function ==
  data: u input; T output
function T = extract_outlet_temps(u)

n=length(u)/2;

u1=u(1:n);
u2=u(n+1:2*n);

T1=u1(end);
T2=u2(end);
T=[T1,T2];
end

== matlab function C_PTES_sim_v2/Hot_side_HXER/MATLAB Function ==
  data: u input; T output
function T = extract_outlet_temps(u)

n=length(u)/2;

u1=u(1:n);
u2=u(n+1:2*n);

T1=u1(end);
T2=u2(end);
T=[T1,T2];
end

== matlab function C_PTES_sim_v2/Air cooler/MATLAB Function1 ==
  data: u input; y output
function y = fcn(u)
if u<0.1
    y=320;
else
    y = 361.15;
end

== matlab function C_PTES_sim_v2/Hot_side_HXER/Average Temperature ==
  data: u input; y output
function y = fcn(u)

n=length(u)/2;

T_CO2= u(1:n);

y = mean(T_CO2);

== matlab function C_PTES_sim_v2/Dryness check (0 for "x<=0" and 1 for "x>=1" i.e. dry) ==
  data: u input; y output
function y = fcn(u)
    if u < 0 && u == 0
        y = 0;
    elseif u > 0 && u < 1
        y = u;
    else
        y = 1;
    end
end

== matlab function C_PTES_sim_v2/Dryness check ==
  data: u input; y output
function y = fcn(u)
    if u < 0 && u == 0
        y = 0;
    elseif u > 0 && u < 1
        y = u;
    else
        y = 1;
    end
end
%% In refprop, 999 indicates superheated and -998 indicates sub cooled

== matlab function C_PTES_sim_v2/Air cooler/Average Temperature ==
  data: u input; y output
function y = fcn(u)

n=length(u)/2;

T_CO2= u(1:n);

y = mean(T_CO2);

== matlab function C_PTES_sim_v2/Recuperator/Average Temperature ==
  data: u input; y output
function y = fcn(u)

n=length(u)/2;

T_CO2_high= u(1:n);
T_CO2_low = u(n+1:2*n);

y = [mean(T_CO2_high) mean(T_CO2_low)];

== matlab function C_PTES_sim_v2/Compressor/Calc Inlet Temp ==
  data: u input; y output
function y = fcn(u)

m_in = u(1);
T_in = u(2);
m_r = u(3);
T_r = u(4);

m_tot = m_in + m_r;

T_comp_in = (m_in*T_in+m_r*T_r)/m_tot;

y = T_comp_in-273.15;

end

== matlab function C_PTES_sim_v2/Compressor/Cool Recycle//Inlet ==
  data: u input; y output
function y = fcn(u)

m_in = u(1);
T_in = u(2);
m_r = u(3);
T_r = u(4);

m_tot = m_in + m_r;

T_comp_in = (m_in*T_in+m_r*T_r)/m_tot;

y = T_comp_in-273.15;

end

== matlab function C_PTES_sim_v2/Compressor/MATLAB Function1 ==
  data: u input; y output; z_v input
function y= fcn(u,z_v)

Valve_in_gain=0.0160055850737664*(1+-7.285480376175610e-05);
In_pres=u(1);
Out_pres=u(2);
m_in     = Valve_in_gain*z_v* sqrt(abs(Out_pres - In_pres)) * (Out_pres - In_pres)/abs(Out_pres - In_pres);
y = m_in;

== matlab function C_PTES_sim_v2/Compressor/MATLAB Function ==
  data: x input; y input
function plotXY(x,y)
%#codegen
    persistent h
    if isempty(h)
        h = figure(4);
        hold on;
    
        % Set fixed limits (change as needed)
        xlim([0 60]);
        ylim([1 3]);
    end
    % Plot new point
    plot(x, y, 'r.');
end

== matlab function C_PTES_sim_v2/Air cooler/MATLAB Function ==
  data: u input; T output
function T = extract_outlet_temps(u)

n=length(u)/2;

u1=u(1:n);
u2=u(n+1:2*n);

T1=u1(end);
T2=u2(end);
T=[T1,T2];
end

== matlab function C_PTES_sim_v2/Compressor/MATLAB Function4 ==
  data: u input; y output
function y = fcn(u)

if u(2)<0.5 && u(3)<0.1

    y = 1;

else
    y=u(1);
end

end
